simulink model "AutosarStructrueTemplete_Harness1"  (R2023b)
settings: Solver=FixedStepDiscrete  StartTime=0.0  StopTime=10.0  FixedStep=0.02  RelTol=1e-3  EnableMultiTasking=on
undefined symbols (not defined in the file): I, initialize, T, terminate
libraries: autosarlibdem x1, autosarlibnvm x1
settings Model: DataDictionary=autosar.sldd  Creator=admin  LastModifiedBy=admin
settings SolverCC: AlgebraicLoopSolver=TrustRegion  AutoInsertRateTranBlk=on  InsertRTBMode=Never (minimum delay)  MaxZcPerStep=1
settings OptimizationCC: DefaultParameterBehavior=Inlined  EnhancedBackFolding=on  PassReuseOutputArgsAs=Individual arguments  ZeroExternalMemoryAtStartup=off  ZeroInternalMemoryAtStartup=off  OptimizeBlockOrder=speed  DifferentSizesBufferReuse=on  OptimizationCustomize=off  EfficientTunableParamExpr=on
settings DebuggingCC: MultiTaskDSMMsg=none  MultiTaskRateTransMsg=warning  ParameterTunabilityLossMsg=error  UnconnectedLineMsg=warning
settings SFSimCC: SimGenImportedTypeDefs=on  MATLABDynamicMemAlloc=off
settings RTWCC: Description=AUTOSAR  SystemTargetFile=autosar.tlc  GenCodeOnly=on  TemplateMakefile=ert_default_tmf  IncludeHyperlinkInReport=on  DataTypeReplacement=CDataTypesFixedWidth  DLArmComputeVersion=19.05
settings CodeAppCC: ForceParamTrailComments=on  IgnoreCustomStorageClasses=off  OperatorAnnotations=on  SimulinkDataObjDesc=on  SFDataObjDesc=on  InsertBlockDesc=on
settings STFCustomTargetCC: MultiwordLength=256  ParMdlRefBuildCompliant=on  CompOptLevelCompliant=on  IncludeMdlTerminateFcn=off  CombineOutputUpdateFcns=on  SuppressErrorStatus=on  ERTCustomFileBanners=on  SupportNonFinite=off  SupportComplex=off  SupportContinuousTime=off  SupportNonInlinedSFcns=off  RemoveResetFunc=on  MATLABClassNameForMDSCustomization=Simulink.SoftwareTarget.ERTCustomization  AutosarCompliant=on  UseToolchainInfoCompliant=on  LookupTableObjectStructAxisOrder=2,1,3,4,...  LUTObjectStructOrderEvenSpacing=Size,Table,Breakpoints  SystemTargetFile=autosar.tlc
settings ERTTargetCC: TargetLangStandard=C99 (ISO)  ConcurrentExecutionCompliant=off  IncludeMdlTerminateFcn=off  SuppressErrorStatus=on  SupportNonFinite=off  SupportComplex=off  ModelStepFunctionPrototypeControlCompliant=off  CPPClassGenCompliant=off  AutosarCompliant=on  LookupTableObjectStructAxisOrder=2,1,3,4,...  LUTObjectStructOrderEvenSpacing=Size,Table,Breakpoints  InlinedParameterPlacement=NonHierarchical  ERTCustomFileTemplate=example_file_process.tlc

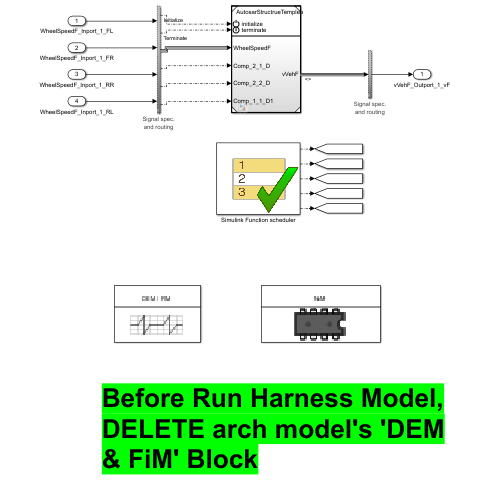
[thumbnail: Simulink's stored preview of the top-level diagram]
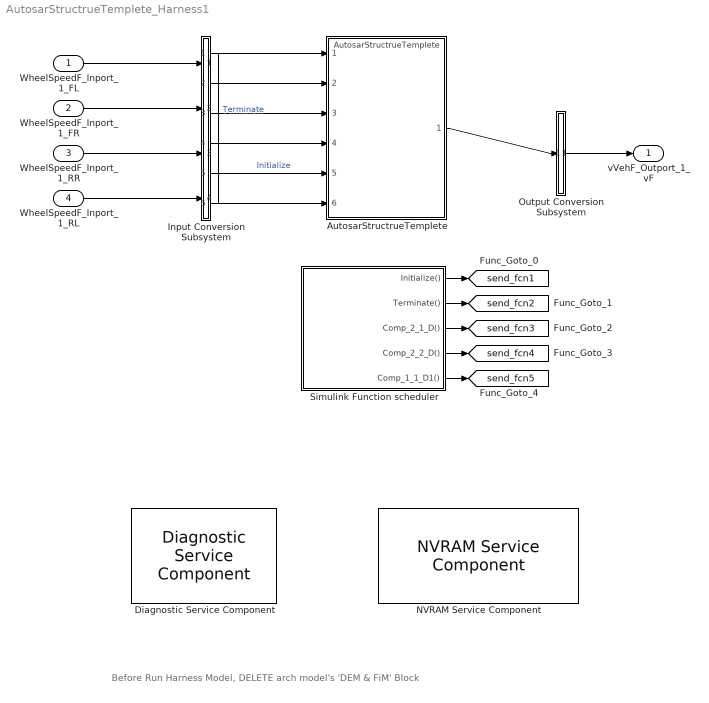
== system AutosarStructrueTemplete_Harness1 ==
  note: Before Run Harness Model, DELETE arch model's 'DEM & FiM' Block
  WheelSpeedF_Inport_1_FL : Inport  OutDataTypeStr=single  PortDimensions=[1]
  WheelSpeedF_Inport_1_FR : Inport  Port=2  OutDataTypeStr=single  PortDimensions=[1]
  WheelSpeedF_Inport_1_RR : Inport  Port=3  OutDataTypeStr=single  PortDimensions=[1]
  WheelSpeedF_Inport_1_RL : Inport  Port=4  OutDataTypeStr=single  PortDimensions=[1]
  AutosarStructrueTemplete : ModelReference  ModelNameDialog=AutosarStructrueTemplete  SimulationMode=Normal  ShowModelInitializePort=on  ShowModelReinitializePorts=on  ShowModelResetPorts=on  ShowModelTerminatePort=on  ScheduleRates=on  ModelEventPortInfo=I:initialize,T:terminate  ModelReferenceVersion=1.33
  Diagnostic Service Component : autosarlibdem/Diagnostic Service Component  Tag=_SLT_SLFunc_Stub_  ClientPortNames={'DiagnosticInfo01'}  ClientPortPortDefinedArguments={'1'}  MaxEventId=10  MaxFID=10  DemDebounceCounterIncrementStepSize=1  DemDebounceCounterDecrementStepSize=1  DemDebounceCounterFailedThreshold=2  DemDebounceCounterPassedThreshold=-1  InhibitionMatrix=[0 0 0 0 0 0 0 0 0 0 0;0 0 0 0 0 0 0 0 0 0 0;0 0 0 0 0 0 0 0 0 0 0;0 0 0 0 0 0 0 0 0 0 0;0 0 0 0 0 0 0 0 0 0 0;0 0 0 0 0 0 0 0 0 0 0;0 0 0 0 0 0 0 0 0 0 0;0 0 0 0 0 0 0 0 0 0 0;0 0 0 0 0 0 0 0 0 0 0;0 0 0 0 0 0 0 0 0 0 0;0 0 0 0 0 0 0 0 0 0 0]  EnableConditionIndexes=zeros(257,'uint8')  StorageConditionIndexes=zeros(257,'uint8')
  Input Conversion Subsystem : Subsystem  Tag=__SLT_ICS__  Description=|
      | Signal spec.
      | and routing
      settings: AttributesFormatString=%<Description>
  NVRAM Service Component : autosarlibnvm/NVRAM Service Component  ClientPortNames={'NvM_Read001'}  ClientPortPortDefinedArguments={'1'}  MaxBlockId=10  NvInitValues={'0'}
  Output Conversion Subsystem : Subsystem  Tag=__SLT_OCS__  Description=|
      | Signal spec.
      | and routing
      settings: AttributesFormatString=%<Description>
  Simulink Function scheduler : Test Sequence  Tag=__SLT_FCN_CALL__  TreatAsAtomicUnit=on
  vVehF_Outport_1_vF : Outport
  tag scope: send_fcn1=global, send_fcn2=global, send_fcn3=global, send_fcn4=global, send_fcn5=global
  wires:
  WheelSpeedF_Inport_1_FL/1 -> Input Conversion Subsystem/1(Inport_1)
  WheelSpeedF_Inport_1_FR/1 -> Input Conversion Subsystem/2(Inport_2)
  WheelSpeedF_Inport_1_RR/1 -> Input Conversion Subsystem/3(Inport_3)
  WheelSpeedF_Inport_1_RL/1 -> Input Conversion Subsystem/4(Inport_4)
  Output Conversion Subsystem/1(Outport_1) -> vVehF_Outport_1_vF/1
  Input Conversion Subsystem/1(Outport_1) -> AutosarStructrueTemplete/5  "Initialize"
  Input Conversion Subsystem/2(Outport_2) -> AutosarStructrueTemplete/6  "Terminate"
  Input Conversion Subsystem/3(Outport_3) -> AutosarStructrueTemplete/1
  Input Conversion Subsystem/4(Outport_4) -> AutosarStructrueTemplete/2
  Input Conversion Subsystem/5(Outport_5) -> AutosarStructrueTemplete/3
  Input Conversion Subsystem/6(Outport_6) -> AutosarStructrueTemplete/4
  AutosarStructrueTemplete/1 -> Output Conversion Subsystem/1(Inport_1)
  Simulink Function scheduler/1(Initialize()) -> [send_fcn1]
  Simulink Function scheduler/2(Terminate()) -> [send_fcn2]
  Simulink Function scheduler/3(Comp_2_1_D()) -> [send_fcn3]
  Simulink Function scheduler/4(Comp_2_2_D()) -> [send_fcn4]
  Simulink Function scheduler/5(Comp_1_1_D1()) -> [send_fcn5]

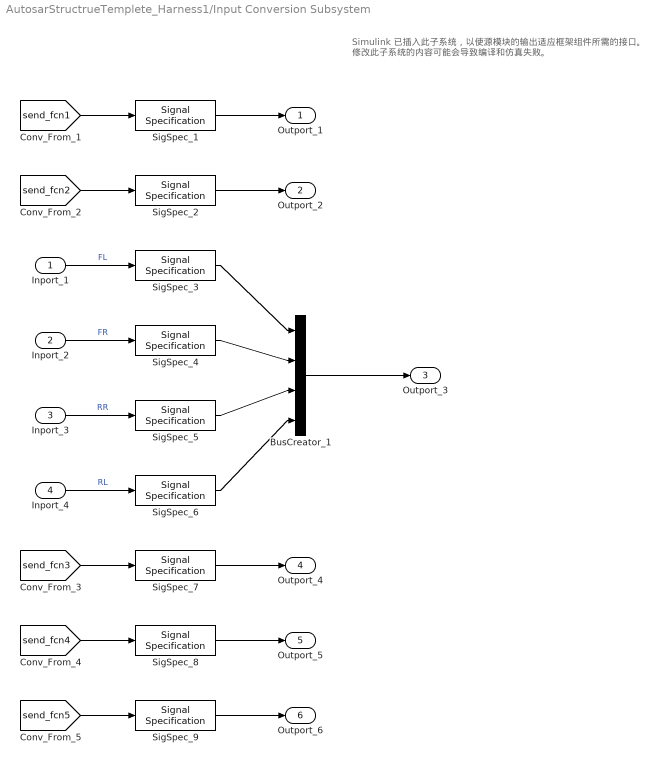
== system AutosarStructrueTemplete_Harness1/Input Conversion Subsystem ==
  note: Simulink 已插入此子系统，以使源模块的输出适应框架组件所需的接口。
      |  修改此子系统的内容可能会导致编译和仿真失败。
  Inport_1 : Inport
  Inport_2 : Inport  Port=2
  Inport_3 : Inport  Port=3
  Inport_4 : Inport  Port=4
  BusCreator_1 : BusCreator  Inputs=4
  SigSpec_{1..2,7..9} (5 alike) : SignalSpecification
  SigSpec_{3..6} (4 alike) : SignalSpecification  OutDataTypeStr=single  Dimensions=[1]
  Outport_1 : Outport
  Outport_2 : Outport  Port=2
  Outport_3 : Outport  Port=3
  Outport_4 : Outport  Port=4
  Outport_5 : Outport  Port=5
  Outport_6 : Outport  Port=6
  wires:
  SigSpec_1/1 -> Outport_1/1
  [send_fcn1] -> SigSpec_1/1
  SigSpec_2/1 -> Outport_2/1
  [send_fcn2] -> SigSpec_2/1
  BusCreator_1/1 -> Outport_3/1
  SigSpec_3/1 -> BusCreator_1/1
  Inport_1/1 -> SigSpec_3/1  "FL"
  SigSpec_4/1 -> BusCreator_1/2
  Inport_2/1 -> SigSpec_4/1  "FR"
  SigSpec_5/1 -> BusCreator_1/3
  Inport_3/1 -> SigSpec_5/1  "RR"
  SigSpec_6/1 -> BusCreator_1/4
  Inport_4/1 -> SigSpec_6/1  "RL"
  SigSpec_7/1 -> Outport_4/1
  [send_fcn3] -> SigSpec_7/1
  SigSpec_8/1 -> Outport_5/1
  [send_fcn4] -> SigSpec_8/1
  SigSpec_9/1 -> Outport_6/1
  [send_fcn5] -> SigSpec_9/1

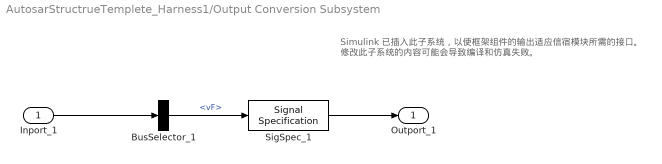
== system AutosarStructrueTemplete_Harness1/Output Conversion Subsystem ==
  note: Simulink 已插入此子系统，以使框架组件的输出适应信宿模块所需的接口。
      |  修改此子系统的内容可能会导致编译和仿真失败。
  Inport_1 : Inport
  BusSelector_1 : BusSelector  OutputSignals=vF
  SigSpec_1 : SignalSpecification  OutDataTypeStr=single  Dimensions=[1]
  Outport_1 : Outport
  wires:
  Inport_1/1 -> BusSelector_1/1
  BusSelector_1/1 -> SigSpec_1/1  "<vF>"
  SigSpec_1/1 -> Outport_1/1

== stateflow chart AutosarStructrueTemplete_Harness1/Simulink Function scheduler ==
  settings: updateMethod=DISCRETE  sampleTime=0.02
  state Run
    %% Call Initialization task.
    if t == 0
    send(Initialize);
    end
    if t == 0 || every(50, tick)
    send(Comp_1_1_D1);
    end
  state AsyncFunctionCalls
    %% Call Asynchronous FunctionCall Subsystems.
    %%
    send(Comp_2_1_D);
    send(Comp_2_2_D);
  state Terminate
    % Call Terminate task.
    % Add transitions to this step as required.
    send(Terminate);
  (default) -> Run
  events: Initialize output FUNCTION_CALL_EVENT; Terminate output FUNCTION_CALL_EVENT; Comp_2_1_D output FUNCTION_CALL_EVENT; Comp_2_2_D output FUNCTION_CALL_EVENT; Comp_1_1_D1 output FUNCTION_CALL_EVENT
